simulink model "Investigation_PMSM"  (R2020a)
settings: Solver=ode3  StartTime=0.0  StopTime=t_end  FixedStep=dt  RelTol=1e-3  EnableMultiTasking=on
settings Model: Creator=julien  LastModifiedBy=ge29wel
settings DataIOCC: LimitDataPoints=on  SaveFormat=Array  ReturnWorkspaceOutputs=off
settings OptimizationCC: ExpressionDepthLimit=2147483647  LifeSpan=inf
settings DebuggingCC: UnderspecifiedInitializationDetection=Classic  MergeDetectMultiDrivingBlocksExec=none  SolverPrmCheckMsg=warning  StateNameClashWarn=warning  SFUnexpectedBacktrackingDiag=warning  SFNoUnconditionalDefaultTransitionDiag=warning  SFExecutionAtInitializationDiag=none  ArithmeticOperatorsInVariantConditions=warning
settings HardwareCC: ProdBitPerPointer=32  ProdBitPerSizeT=32  ProdBitPerPtrDiffT=32  ProdLargestAtomicFloat=None  ProdIntDivRoundTo=Undefined  ProdEndianess=Unspecified  ProdWordSize=32  ProdHWDeviceType=32-bit Generic
settings ModelReferenceCC: PropagateSignalLabelsOutOfModel=off
settings SFSimCC: SimUseLocalCustomCode=off  CustomCodeUndefinedFunction=UseInterfaceOnly
settings RTWCC: RTWUseLocalCustomCode=off
settings CodeAppCC: StateflowObjectComments=on
settings GRTTargetCC: TargetLangStandard=C89/C90 (ANSI)
settings ConfigComp: CovMetricSettings=dw  CovHtmlReporting=on  CovSaveCumulativeToWorkspaceVar=on  CovSaveSingleToWorkspaceVar=on  CovExternalEMLEnable=off  CovSFcnEnable=off

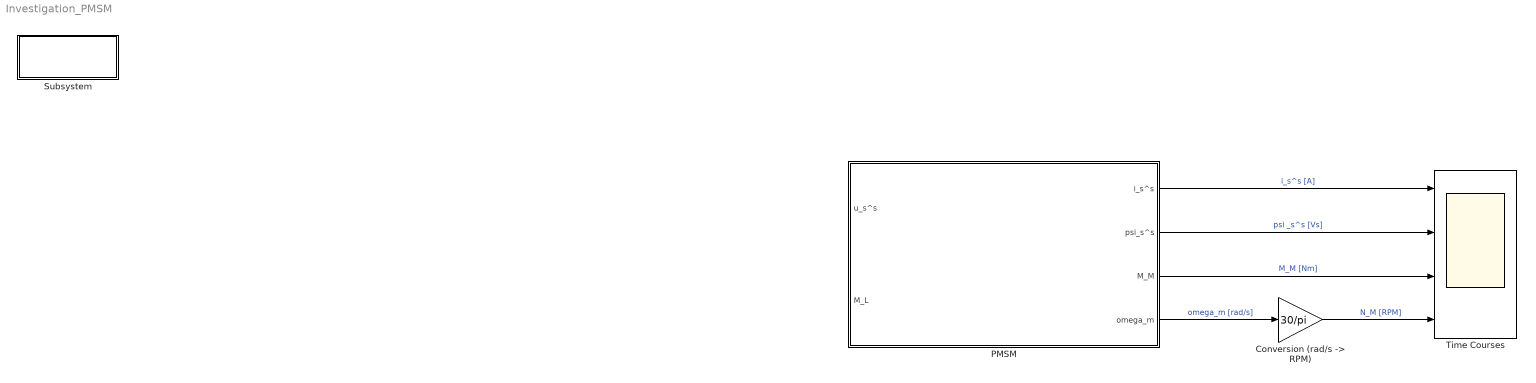
== system Investigation_PMSM ==
  "Conversion (rad/s -> RPM)" : Gain  Gain=30/pi
  PMSM : Subsystem
  Subsystem : Subsystem
      settings: OpenFcn=Experiment_3_PMSM_Parameter
      mask Display: disp('Initialize\n (doppelklicken)')
  Time Courses : Scope  NumInputPorts=4
  wires:
  PMSM/3(M_M) -> Time Courses/3  "M_M [Nm]"
  PMSM/1(i_s^s) -> Time Courses/1  "i_s^s [A]"
  PMSM/4(omega_m) -> "Conversion (rad/s -> RPM)"/1  "omega_m [rad/s]"
  "Conversion (rad/s -> RPM)"/1 -> Time Courses/4  "N_M [RPM]"
  PMSM/2(psi_s^s) -> Time Courses/2  "psi _s^s [Vs]"

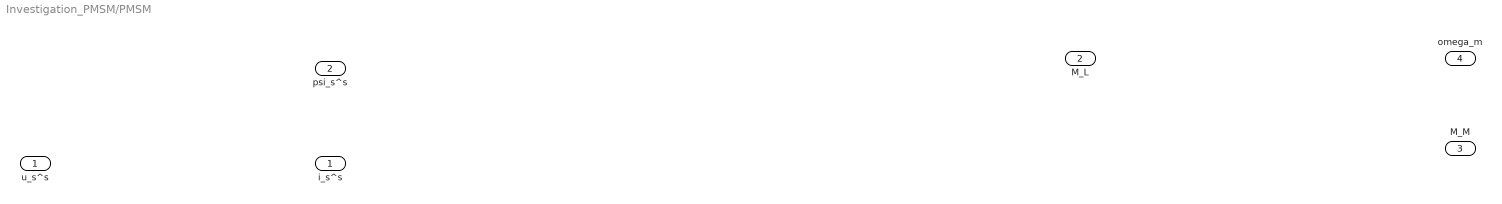
== system Investigation_PMSM/PMSM ==
  u_s^s : Inport
  M_L : Inport  Port=2
  i_s^s : Outport
  psi_s^s : Outport  Port=2
  M_M : Outport  Port=3
  omega_m : Outport  Port=4

== system Investigation_PMSM/Subsystem ==
